simulink model "BD_FUELCELL"  (Simulink 7.9)
settings: Solver=ode1  SolverMode=SingleTasking  StartTime=0.0  StopTime=max(cyc_mph(:,1))  FixedStep=1  MaxStep=1  RelTol=1e-3  AbsTol=1e-3
undefined symbols (not defined in the file): ex_calc, fc_emis
libraries: lib_wheel x2, lib_controls x2, lib_help x2, lib_transmission x2, lib_outputs x1, lib_interactive x1, lib_drive_cycle x1, lib_accessory x1, lib_energy_storage x1, lib_exhaust x1, lib_fuel_cell x1, lib_electric_machine x1
settings Model: Creator=mokeefe  LastModifiedBy=mokeefe  ExtModeTrigMode=oneshot  ExtModeArmWhenConnect=off
settings Model: ModifiedComment=|
  | mokeefe -- Fri Mar 23 15:51:49 2012 -- Version 1.79
  | Upgrade parameterized links and upgrade file to latest Simulink.
settings Model: ModifiedHistory=|
  | mokeefe -- Fri Mar 23 15:51:49 2012 -- Version 1.79
  | Upgrade parameterized links and upgrade file to latest Simulink.
  | 
  | ssprik -- Wed Sep 24 14:55:17 2003 -- Version 1.78
  | 
  | 
  | kharalds -- Tue Jun 10 10:04:01 2003 -- Version 1.77
  | undid the prior change (back to 10000) in Fuel Cell Power System Model/min_cell_voltage & net power gen/algebraic constraint/initial guess
  | 
  | kharalds -- Tue Jun 10 09:48:54 2003 -- Version 1.76
  | in Fuel Cell Power System Model/min_cell_voltage & net power gen/algebraic constraint/Initial guess: changed value from 40000 to 10000.
  | 
  | bjeanner -- Tue Dec 10 15:48:38 2002 -- Version 1.75
  | 
  | 
  | bjeanner -- Tue Dec 10 15:20:32 2002 -- Version 1.74
  | 
  | 
  | bjeanner -- Tue Dec 10 11:52:09 2002 -- Version 1.73
  | 
  | 
  | bjeanner -- Tue Dec 10 11:30:33 2002 -- Version 1.72
  | 
  | 
  | bjeanner -- Tue Dec 10 11:22:18 2002 -- Version 1.71
  | 
  | 
  | bjeanner -- Tue Dec 10 11:18:18 2002 -- Version 1.70
  | 
  | 
  | bjeanner -- Tue Dec 10 10:31:06 2002 -- Version 1.69
  | 
  | 
  | bjeanner -- Tue Dec 10 10:30:27 2002 -- Version 1.68
  | 
  | 
  | bjeanner -- Tue Dec 10 10:23:40 2002 -- Version 1.67
  | 
  | 
  | tmarkel -- Fri Sep 06 14:56:54 2002 -- Version 1.66
  | VT and KTH fuel cell models in place
  | 
  | 
  | tmarkel -- Fri Sep 06 12:17:07 2002 -- Version 1.65
  | akfd
  | 
  | 
  | tmarkel -- Fri Sep 06 11:53:29 2002 -- Version 1.64
  | replaced bad link to altia with link to interactive library block
  | 
  | 
  | tmarkel -- Mon Aug 12 17:09:32 2002 -- Version 1.63
  | trying to get it to see the cinfig sys names
  | 
  | ssprik -- Mon Apr 22 11:29:38 2002 -- Version 1.62
  | 
  | 
  | ssprik -- Mon Apr 22 11:22:32 2002 -- Version 1.61
  | 
  | 
  | ssprik -- Mon Apr 22 11:21:51 2002 -- Version 1.60
  | 
  | 
  | tmarkel -- Sat Apr 20 11:16:25 2002 -- Version 1.59
  | replaced fuel cell linked library model with config system model
  | 
  | 
  | mokeefe -- Thu Apr 18 07:55:48 2002 -- Version 1.58
  | saving the model:
  | o "without the model browser open"
  | o with only top-level screen visible
  | o and with "fit to view" enabled
  | 
  | mokeefe -- Thu Apr 18 07:45:26 2002 -- Version 1.57
  | saving the model:
  | o "without the model browser open"
  | o with only top-level screen visible
  | o and with "fit to view" enabled
settings DataIOCC: LimitDataPoints=off  SaveOutput=off  SaveTime=off
settings OptimizationCC: BooleanDataType=off
settings DebuggingCC: SaveWithParameterizedLinksMsg=none  SignalResolutionControl=TryResolveAllWithWarning  SolverPrmCheckMsg=none  MultiTaskDSMMsg=warning  MultiTaskCondExecSysMsg=none  UnconnectedLineMsg=none  StrictBusMsg=None
settings HardwareCC: TargetUnknown=on
settings RTWCC: TemplateMakefile=grt_vc.tmf  IncludeERTFirstTime=on
settings GRTTargetCC: CombineOutputUpdateFcns=off  GRTInterface=on

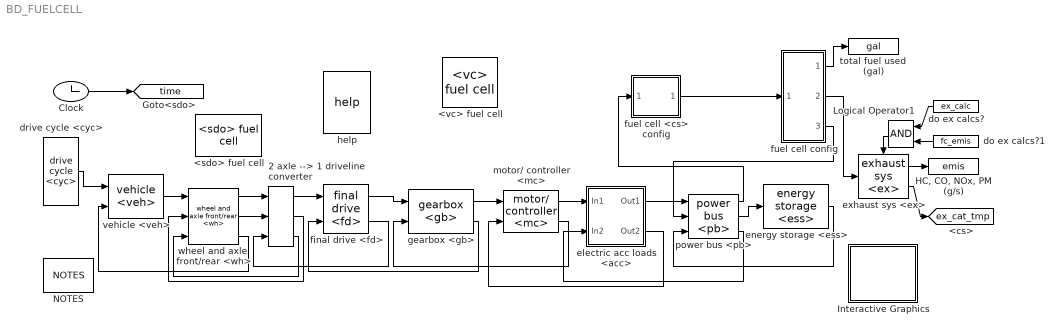
== system BD_FUELCELL ==
  2 axle --> 1 driveline converter : lib_wheel/2 axle --> 1 driveline converter
  <sdo> fuel cell : lib_outputs/<sdo> fuel cell  SystemSampleTime=-1
  <vc> fuel cell : lib_controls/<vc> fuel cell  SystemSampleTime=-1
  Clock : Clock
  "HC, CO, NOx, PM (g/s)" : ToWorkspace  VariableName=emis
  Interactive Graphics : Subsystem  BlockChoice=off
      link override off/Live Inputs/veh/roll res interactive: BlockChoice=roll res force req (N)
      settings: AttributesFormatString=%<BlockChoice>  TemplateBlock=lib_interactive/Interactive Graphics  MemberBlocks=off,on
  Logical Operator1 : Logic
  NOTES : lib_help/NOTES  SystemSampleTime=-1
  do ex calcs? : Constant  Value=ex_calc
  do ex calcs?1 : Constant  Value=fc_emis
  drive cycle <cyc> : lib_drive_cycle/drive cycle <cyc>  SystemSampleTime=-1
  electric acc loads <acc> : Subsystem
      mask Display: image(imread('bdi_acc_elec.bmp'))
  energy storage <ess> : lib_energy_storage/energy storage <ess>  SystemSampleTime=-1
  exhaust sys <ex> : lib_exhaust/exhaust sys <ex>  SystemSampleTime=-1
  final drive <fd> : lib_transmission/final drive <fd>  SystemSampleTime=-1
  fuel cell <cs> config : Subsystem  BlockChoice=fuel cell control strategy <cs>
      settings: AttributesFormatString=%<BlockChoice>  TemplateBlock=lib_controls/fuel cell <cs> config  MemberBlocks=fuel cell adaptive <cs>,fuel cell control strategy <cs>
  fuel cell config : Subsystem  BlockChoice=fuel converter <fc> VT model
      link override fuel converter <fc> VT model/Fuel Cell Power System Model (S. Gurski - Virgina Tech)/min_cell_voltage & net power gen/Algebraic Constraint1: z0=40000
      settings: AttributesFormatString=%<BlockChoice>  TemplateBlock=lib_fuel_cell/fuel cell config  MemberBlocks="fuel converter <fc>  KTH fc model,fuel converter <fc> GCTool linkage,fuel converter <fc> VT model,fuel converter <fc> net model,fuel converter <fc> polarization curve model"
  gearbox <gb> : lib_transmission/gearbox <gb>  SystemSampleTime=-1
  help : lib_help/help  SystemSampleTime=-1
  motor/ controller <mc> : lib_electric_machine/motor// controller <mc>  SystemSampleTime=-1
  power bus <pb> : lib_power_bus/power bus <pb>  SystemSampleTime=-1
  total fuel used  (gal) : ToWorkspace  VariableName=gal
  vehicle <veh> : lib_vehicle/vehicle <veh>  SystemSampleTime=-1
  wheel and axle  front/rear <wh> : lib_wheel/wheel and axle  front//rear <wh>  SystemSampleTime=-1
  tag scope: ex_cat_tmp=global, time=global
  wires:
  final drive <fd>/2 -> 2 axle --> 1 driveline converter/3
  2 axle --> 1 driveline converter/1 -> final drive <fd>/1
  wheel and axle  front/rear <wh>/3 -> vehicle <veh>/2
  final drive <fd>/1 -> gearbox <gb>/1
  drive cycle <cyc>/1 -> vehicle <veh>/1
  Clock/1 -> [time]
  energy storage <ess>/1 -> power bus <pb>/3
  power bus <pb>/2 -> energy storage <ess>/1
  motor/ controller <mc>/2 -> gearbox <gb>/2
  gearbox <gb>/1 -> motor/ controller <mc>/1
  gearbox <gb>/2 -> final drive <fd>/2
  power bus <pb>/1 -> fuel cell <cs> config/1(power req'd by bus (W))
  fuel cell <cs> config/1(engine pwr (W)) -> fuel cell config/1(pwr req'd at fc  output (W))
  fuel cell config/2(EO emis info) -> exhaust sys <ex>/1
  fuel cell config/1(fuel use) -> total fuel used  (gal)/1
  do ex calcs?/1 -> Logical Operator1/1
  exhaust sys <ex>/1 -> "HC, CO, NOx, PM (g/s)"/1
  Logical Operator1/1 -> exhaust sys <ex>/Enable
  do ex calcs?1/1 -> Logical Operator1/2
  fuel cell config/3(pwr avail. to driveline (W)) -> power bus <pb>/2
  exhaust sys <ex>/2 -> [ex_cat_tmp]
  motor/ controller <mc>/1 -> electric acc loads <acc>/1(In1)
  electric acc loads <acc>/1(Out1) -> power bus <pb>/1
  power bus <pb>/3 -> electric acc loads <acc>/2(In2)
  electric acc loads <acc>/2(Out2) -> motor/ controller <mc>/2
  wheel and axle  front/rear <wh>/1 -> 2 axle --> 1 driveline converter/1
  wheel and axle  front/rear <wh>/2 -> 2 axle --> 1 driveline converter/2
  2 axle --> 1 driveline converter/2 -> wheel and axle  front/rear <wh>/2
  2 axle --> 1 driveline converter/3 -> wheel and axle  front/rear <wh>/3
  vehicle <veh>/1 -> wheel and axle  front/rear <wh>/1

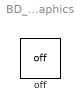
== system BD_FUELCELL/Interactive Graphics ==
  off : lib_interactive/off  Tag=Altia_off  SystemSampleTime=-1

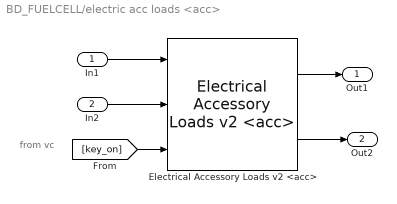
== system BD_FUELCELL/electric acc loads <acc> ==
  note: from vc
  In1 : Inport
  In2 : Inport  Port=2
  Electrical Accessory Loads v2 <acc> : lib_accessory/Electrical Accessory Loads v2 <acc>  load_on=1
  Out1 : Outport
  Out2 : Outport  Port=2
  wires:
  In1/1 -> Electrical Accessory Loads v2 <acc>/1
  In2/1 -> Electrical Accessory Loads v2 <acc>/2
  Electrical Accessory Loads v2 <acc>/1 -> Out1/1
  Electrical Accessory Loads v2 <acc>/2 -> Out2/1
  [key_on] -> Electrical Accessory Loads v2 <acc>/3

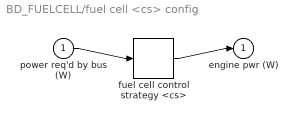
== system BD_FUELCELL/fuel cell <cs> config ==
  power req'd by bus (W) : Inport
  fuel cell control strategy <cs> : lib_controls/fuel cell control strategy <cs>  SystemSampleTime=-1
  engine pwr (W) : Outport
  wires:
  power req'd by bus (W)/1 -> fuel cell control strategy <cs>/1
  fuel cell control strategy <cs>/1 -> engine pwr (W)/1

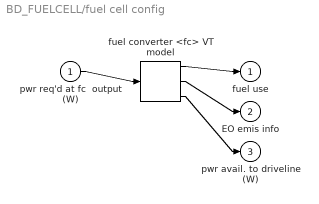
== system BD_FUELCELL/fuel cell config ==
  pwr req'd at fc  output (W) : Inport
  fuel converter <fc> VT model : lib_fuel_cell/fuel converter <fc> VT model  SystemSampleTime=-1
  fuel use : Outport
  EO emis info : Outport  Port=2
  pwr avail. to driveline (W) : Outport  Port=3
  wires:
  pwr req'd at fc  output (W)/1 -> fuel converter <fc> VT model/1
  fuel converter <fc> VT model/1 -> fuel use/1
  fuel converter <fc> VT model/2 -> EO emis info/1
  fuel converter <fc> VT model/3 -> pwr avail. to driveline (W)/1
